simulink model "rpi_simulink_demo_flight"  (R2016b)
settings: Solver=FixedStepAuto  StartTime=0.0  StopTime=inf  MaxStep=0.001  RelTol=1e-3
undefined symbols (not defined in the file or in its folder): rpi_in, rpi_out
settings Model: Creator=Patrick  LastModifiedBy=Patrick
settings SolverCC: PositivePriorityOrder=on
settings OptimizationCC: MaxStackSize=64
settings DebuggingCC: ParameterTunabilityLossMsg=error
settings HardwareCC: ProdBitPerPointer=32  ProdBitPerSizeT=32  ProdBitPerPtrDiffT=32  ProdLargestAtomicInteger=Long  ProdLargestAtomicFloat=Double  ProdWordSize=32  ProdHWDeviceType=ARM Compatible->ARM Cortex  UseEmbeddedCoderFeatures=off  UseSimulinkCoderFeatures=off
settings RTWCC: SystemTargetFile=ert.tlc  HardwareBoard=Raspberry Pi  TLCOptions="-aInlineSetEventsForThisBaseRateFcn=TLC_FALSE -aSuppressMultiTaskScheduler=TLC_FALSE  -aRateBasedStepFcn=0"  TemplateMakefile=ert_default_tmf  Description=Embedded Coder  GenerateReport=on  Toolchain=GNU GCC Raspberry Pi  LaunchReport=on
settings CodeAppCC: ForceParamTrailComments=on  OperatorAnnotations=on  MATLABSourceComments=on
settings ERTTargetCC: ERTCustomFileBanners=off  SupportContinuousTime=on  SupportNonInlinedSFcns=on  RemoveResetFunc=off  SupportVariableSizeSignals=on  ModelStepFunctionPrototypeControlCompliant=off

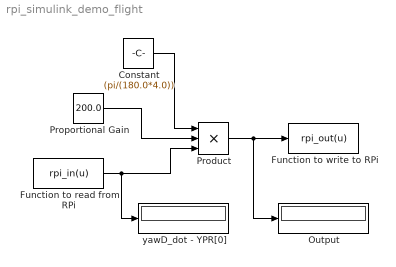
== system rpi_simulink_demo_flight ==
  Constant : Constant  Value=(pi/(180.0*4.0))
  Function to read from RPi : MATLABFcn  MATLABFcn=rpi_in(u)
  Function to write to RPi : MATLABFcn  MATLABFcn=rpi_out(u)
  Output : Display
  Product : Product  Inputs=3
  Proportional Gain : Constant  Value=200.0
  yawD_dot - YPR[0] : Display
  wires:
  Constant/1 -> Product/1
  Proportional Gain/1 -> Product/2
  Function to read from RPi/1 -> yawD_dot - YPR[0]/1, Product/3
  Product/1 -> Function to write to RPi/1, Output/1
